simulink model "signalFilter_ver"  (R2019a)
settings: Solver=VariableStepAuto  StartTime=0.0  StopTime=(nSamp - 1)*Ts  RelTol=1e-3
InitFcn:
  | block_verScript;
StopFcn:
  | filtTestStop;
values from neighbouring files (symbols this model uses):
  FFT_size = 64    [FIR_filterTestm.m]    (also in JMAP_INIT.m; blockVerification.m; block_verScript.m; ksi_verScript.m)
  Ts = 1/Fs    (= 2.08333333333e-05)    [FIR_filterTestm.m]    (also in JMAP_INIT.m; blockVerification.m; block_verScript.m; ksi_verScript.m)
libraries: simulink x3, dsphdlfiltering x3, hdlsllib x2
settings Model: Creator=Showi  LastModifiedBy=Showi

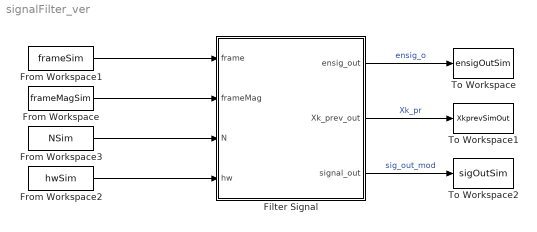
== system signalFilter_ver ==
  Filter Signal : Subsystem
  From Workspace : FromWorkspace  VariableName=frameMagSim  SampleTime=Ts
  From Workspace1 : FromWorkspace  VariableName=frameSim  SampleTime=Ts
  From Workspace2 : FromWorkspace  VariableName=hwSim  SampleTime=Ts
  From Workspace3 : FromWorkspace  VariableName=NSim  SampleTime=Ts
  To Workspace : ToWorkspace  VariableName=ensigOutSim  SaveFormat=Timeseries  SampleTime=-1
  To Workspace1 : ToWorkspace  VariableName=XkprevSimOut  SaveFormat=Timeseries  SampleTime=-1
  To Workspace2 : ToWorkspace  VariableName=sigOutSim  SaveFormat=Timeseries  SampleTime=-1
  wires:
  From Workspace/1 -> Filter Signal/2(frameMag)
  From Workspace1/1 -> Filter Signal/1(frame)
  From Workspace3/1 -> Filter Signal/3(N)
  From Workspace2/1 -> Filter Signal/4(hw)
  Filter Signal/1(ensig_out) -> To Workspace/1  "ensig_o"
  Filter Signal/2(Xk_prev_out) -> To Workspace1/1  "Xk_pr"
  Filter Signal/3(signal_out) -> To Workspace2/1  "sig_out_mod"

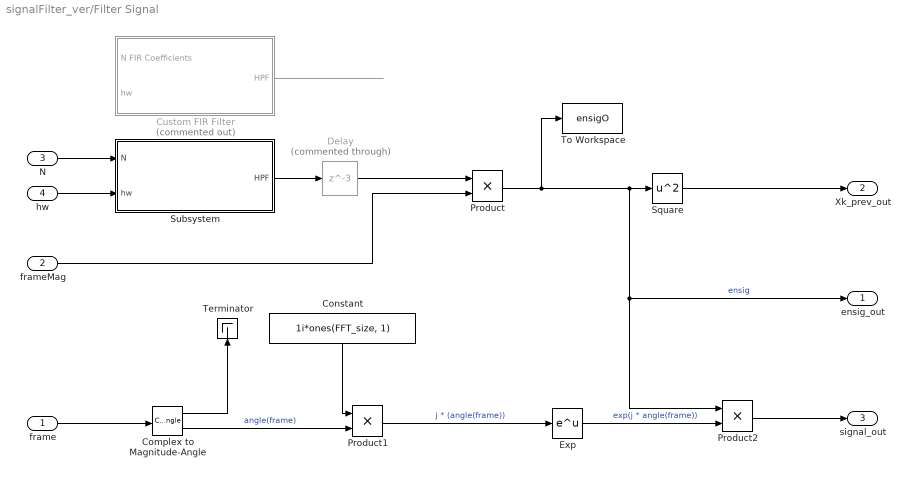
== system signalFilter_ver/Filter Signal ==
  frame : Inport
  frameMag : Inport  Port=2
  N : Inport  Port=3
  hw : Inport  Port=4
  Complex to Magnitude-Angle : ComplexToMagnitudeAngle
  Constant : Constant  Value=1i*ones(FFT_size, 1)  SampleTime=-1
  Custom FIR Filter : Subsystem  Commented=on
  Delay : Delay  Commented=through  DelayLength=3
  Exp : Math  SaturateOnIntegerOverflow=on
  Product : Product
  Product1 : Product
  Product2 : Product
  Square : Math  Operator=square  RndMeth=Zero  SaturateOnIntegerOverflow=on
  Subsystem : Subsystem
  Terminator : Terminator
  To Workspace : ToWorkspace  VariableName=ensigO  SaveFormat=Structure With Time  SampleTime=-1
  ensig_out : Outport
  Xk_prev_out : Outport  Port=2
  signal_out : Outport  Port=3
  wires:
  Square/1 -> Xk_prev_out/1
  frameMag/1 -> Product/2
  Product1/1 -> Exp/1  "j * (angle(frame))"
  Constant/1 -> Product1/1
  Exp/1 -> Product2/2  "exp(j * angle(frame))"
  Product2/1 -> signal_out/1
  Complex to Magnitude-Angle/2 -> Product1/2  "angle(frame)"
  Complex to Magnitude-Angle/1 -> Terminator/1
  N/1 -> Subsystem/1(N)
  hw/1 -> Subsystem/2(hw)
  frame/1 -> Complex to Magnitude-Angle/1
  Product/1 -> To Workspace/1, ensig_out/1, Product2/1, Square/1  "ensig"
  Custom FIR Filter/1(HPF) -> ?
  Subsystem/1(HPF) -> Delay/1
  Delay/1 -> Product/1

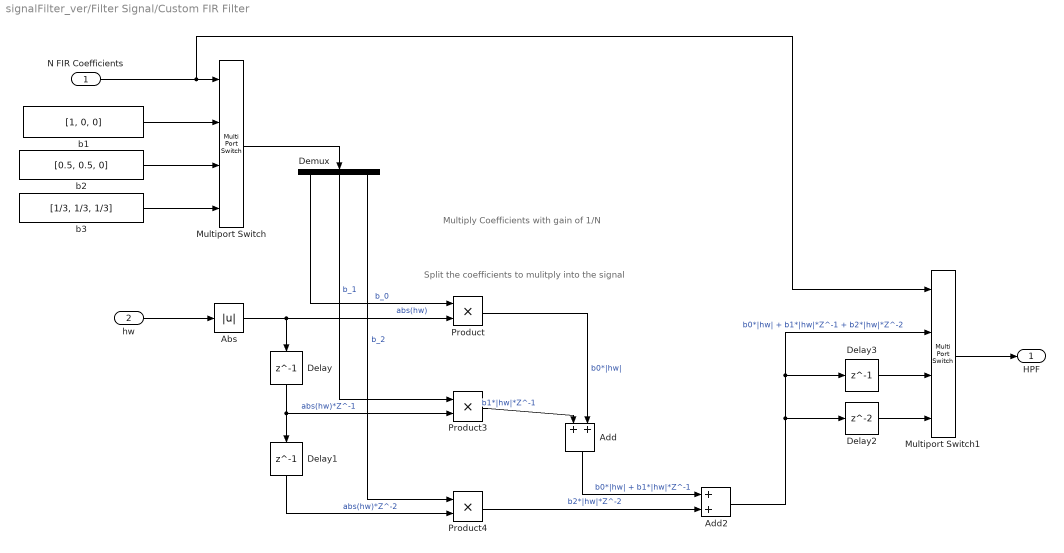
== system signalFilter_ver/Filter Signal/Custom FIR Filter ==
  note: Split the coefficients to mulitply into the signal
  note: Multiply Coefficients with gain of 1/N
  N FIR Coefficients : Inport
  hw : Inport  Port=2
  Abs : Abs
  Add : Sum
  Add2 : Sum
  Delay : Delay  DelayLength=1
  Delay1 : Delay  DelayLength=1
  Delay2 : Delay
  Delay3 : Delay  DelayLength=1
  Demux : Demux  Outputs=3
  Multiport Switch : MultiPortSwitch  DiagnosticForDefault=Warning
  Multiport Switch1 : MultiPortSwitch  DiagnosticForDefault=Warning
  Product : Product
  Product3 : Product
  Product4 : Product
  b1 : Constant  Value=[1, 0, 0]  SampleTime=-1
  b2 : Constant  Value=[0.5, 0.5, 0]  SampleTime=-1
  b3 : Constant  Value=[1/3, 1/3, 1/3]  SampleTime=-1
  HPF : Outport
  wires:
  Delay/1 -> Delay1/1, Product3/2  "abs(hw)*Z^-1"
  Product/1 -> Add/2  "b0*|hw|"
  Product3/1 -> Add/1  "b1*|hw|*Z^-1"
  Abs/1 -> Product/2, Delay/1  "abs(hw)"
  Product4/1 -> Add2/2  "b2*|hw|*Z^-2"
  hw/1 -> Abs/1
  Delay1/1 -> Product4/2  "abs(hw)*Z^-2"
  Add/1 -> Add2/1  "b0*|hw| + b1*|hw|*Z^-1"
  Add2/1 -> Multiport Switch1/2, Delay3/1, Delay2/1  "b0*|hw| + b1*|hw|*Z^-1 + b2*|hw|*Z^-2"
  Demux/1 -> Product/1  "b_0"
  Demux/2 -> Product3/1  "b_1"
  Demux/3 -> Product4/1  "b_2"
  b1/1 -> Multiport Switch/2
  b2/1 -> Multiport Switch/3
  b3/1 -> Multiport Switch/4
  Multiport Switch/1 -> Demux/1
  N FIR Coefficients/1 -> Multiport Switch1/1, Multiport Switch/1
  Delay3/1 -> Multiport Switch1/3
  Delay2/1 -> Multiport Switch1/4
  Multiport Switch1/1 -> HPF/1

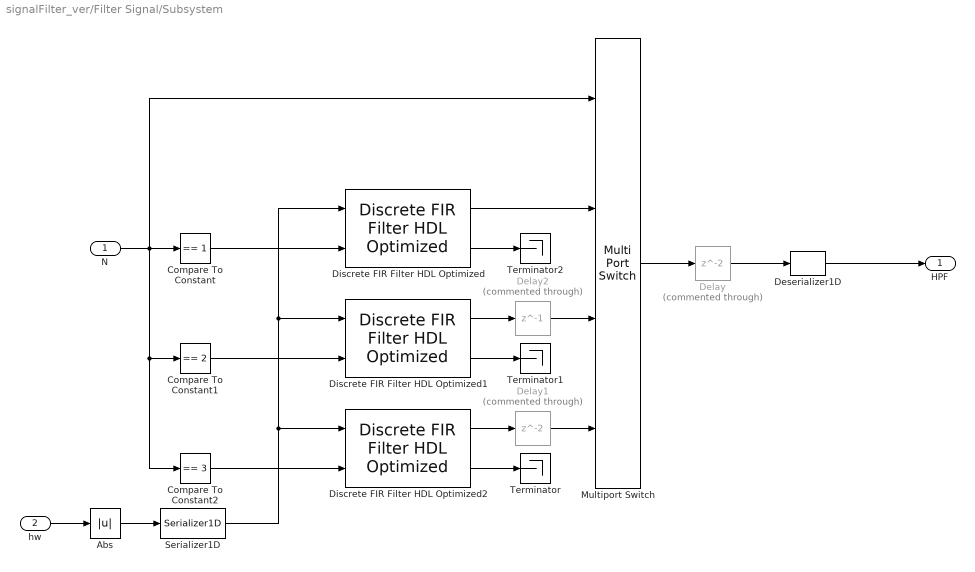
== system signalFilter_ver/Filter Signal/Subsystem ==
  N : Inport
  hw : Inport  Port=2
  Abs : Abs
  Compare To Constant : simulink/Logic and Bit Operations/Compare To Constant  relop===  const=1  OutDataTypeStr=boolean
  Compare To Constant1 : simulink/Logic and Bit Operations/Compare To Constant  relop===  const=2  OutDataTypeStr=boolean
  Compare To Constant2 : simulink/Logic and Bit Operations/Compare To Constant  relop===  const=3  OutDataTypeStr=boolean
  Delay : Delay  Commented=through
  Delay1 : Delay  Commented=through
  Delay2 : Delay  Commented=through  DelayLength=1
  Deserializer1D : hdlsllib/HDL Operations/Deserializer1D  Ratio=FFT_size  IdleCycles=0  InitialCondition=0  startIn=off  validIn=off  validOut=off  inputDataDimensions=-1  inputSampleTime=-1  inputSignalType=auto
      settings: SourceProductName=Simulink  SourceProductBaseCode=SL
  Discrete FIR Filter HDL Optimized : dsphdlfiltering/Discrete FIR Filter HDL Optimized  NumeratorSource=Property  Numerator=[1, 0, 0]  NumeratorPrototype=[ 0.5, 0.5 ]  FilterStructure=Direct form systolic  SerializationOption=Minimum number of cycles between valid input samples  NumberOfCycles=2  NumberOfMultipliers=2  SimulateUsing=Code generation  roundingMode=Floor  overflowMode=off  CoefficientsDataTypeStr=Inherit: Same word length as input  CoefficientsMin=[]  CoefficientsMax=[]  OutputMin=[]  OutputMax=[]  ResetInputPort=off  HDLGlobalReset=off
      settings: SourceProductName=DSP System Toolbox  SourceProductBaseCode=DS
  Discrete FIR Filter HDL Optimized1 : dsphdlfiltering/Discrete FIR Filter HDL Optimized  NumeratorSource=Property  Numerator=[1/2, 1/2, 0]  NumeratorPrototype=[ 0.5, 0.5 ]  FilterStructure=Direct form systolic  SerializationOption=Minimum number of cycles between valid input samples  NumberOfCycles=2  NumberOfMultipliers=2  SimulateUsing=Code generation  roundingMode=Floor  overflowMode=off  CoefficientsDataTypeStr=Inherit: Same word length as input  CoefficientsMin=[]  CoefficientsMax=[]  OutputMin=[]  OutputMax=[]  ResetInputPort=off  HDLGlobalReset=off
      settings: SourceProductName=DSP System Toolbox  SourceProductBaseCode=DS
  Discrete FIR Filter HDL Optimized2 : dsphdlfiltering/Discrete FIR Filter HDL Optimized  NumeratorSource=Property  Numerator=[1/3, 1/3, 1/3]  NumeratorPrototype=[ 0.5, 0.5 ]  FilterStructure=Direct form systolic  SerializationOption=Minimum number of cycles between valid input samples  NumberOfCycles=2  NumberOfMultipliers=2  SimulateUsing=Code generation  roundingMode=Floor  overflowMode=off  CoefficientsDataTypeStr=Inherit: Same word length as input  CoefficientsMin=[]  CoefficientsMax=[]  OutputMin=[]  OutputMax=[]  ResetInputPort=off  HDLGlobalReset=off
      settings: SourceProductName=DSP System Toolbox  SourceProductBaseCode=DS
  Multiport Switch : MultiPortSwitch
  Serializer1D : hdlsllib/HDL Operations/Serializer1D  Ratio=FFT_size  IdleCycles=0  validIn=off  startOut=off  validOut=off  inputDataDimensions=-1  inputSampleTime=-1  inputSignalType=auto
      settings: SourceProductName=Simulink  SourceProductBaseCode=SL
  Terminator : Terminator
  Terminator1 : Terminator
  Terminator2 : Terminator
  HPF : Outport
  wires:
  N/1 -> Multiport Switch/1, Compare To Constant2/1, Compare To Constant1/1, Compare To Constant/1
  hw/1 -> Abs/1
  Compare To Constant/1 -> Discrete FIR Filter HDL Optimized/2
  Compare To Constant1/1 -> Discrete FIR Filter HDL Optimized1/2
  Compare To Constant2/1 -> Discrete FIR Filter HDL Optimized2/2
  Abs/1 -> Serializer1D/1
  Discrete FIR Filter HDL Optimized/1 -> Multiport Switch/2
  Discrete FIR Filter HDL Optimized1/1 -> Delay2/1
  Discrete FIR Filter HDL Optimized2/1 -> Delay1/1
  Multiport Switch/1 -> Delay/1
  Discrete FIR Filter HDL Optimized2/2 -> Terminator/1
  Discrete FIR Filter HDL Optimized1/2 -> Terminator1/1
  Discrete FIR Filter HDL Optimized/2 -> Terminator2/1
  Serializer1D/1 -> Discrete FIR Filter HDL Optimized/1, Discrete FIR Filter HDL Optimized1/1, Discrete FIR Filter HDL Optimized2/1
  Deserializer1D/1 -> HPF/1
  Delay/1 -> Deserializer1D/1
  Delay1/1 -> Multiport Switch/4
  Delay2/1 -> Multiport Switch/3
